simulink model "LazoAbierto_ConROS"  (R2021b)
settings: Solver=FixedStepAuto  StartTime=0.0  StopTime=8  FixedStep=T  RelTol=1e-3
undefined symbols (not defined in the file): fze, ModelName, Pose, ReferenceFrame, T, Twist
libraries: robotlib x13, robotcorelib x1
settings Model: Creator=carlo  LastModifiedBy=carlo
settings OptimizationCC: EnhancedBackFolding=on  PassReuseOutputArgsAs=Individual arguments  ZeroExternalMemoryAtStartup=off  ZeroInternalMemoryAtStartup=off  MaxStackSize=64  OptimizeBlockOrder=speed  DifferentSizesBufferReuse=on  OptimizationCustomize=off  EfficientTunableParamExpr=on
settings DebuggingCC: ParameterTunabilityLossMsg=error
settings HardwareCC: ProdBitPerLong=64  ProdHWDeviceType=Intel->x86-64 (Linux 64)  UseEmbeddedCoderFeatures=off
settings SFSimCC: MATLABDynamicMemAlloc=off
settings RTWCC: Description=Embedded Coder  SystemTargetFile=ert.tlc  HardwareBoard=Robot Operating System (ROS)  TLCOptions="-aInlineSetEventsForThisBaseRateFcn=TLC_FALSE -aSuppressMultiTaskScheduler=TLC_FALSE  -aRateBasedStepFcn=0"  TemplateMakefile=ert_default_tmf  Toolchain=Catkin  TargetLang=C++
settings CodeAppCC: ForceParamTrailComments=on  IgnoreCustomStorageClasses=off  OperatorAnnotations=on  SimulinkDataObjDesc=on  SFDataObjDesc=on  InsertBlockDesc=on
settings ERTTargetCC: SupportNonInlinedSFcns=on

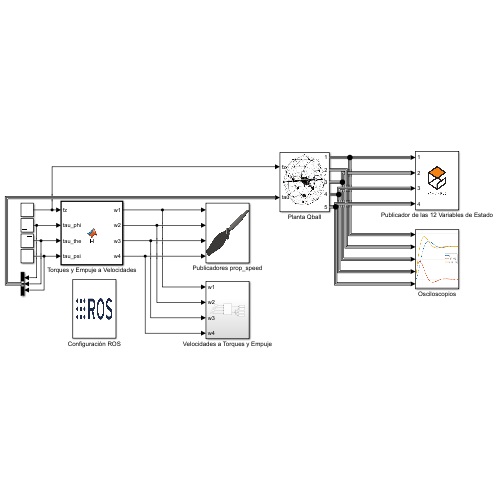
[thumbnail: Simulink's stored preview of the top-level diagram]
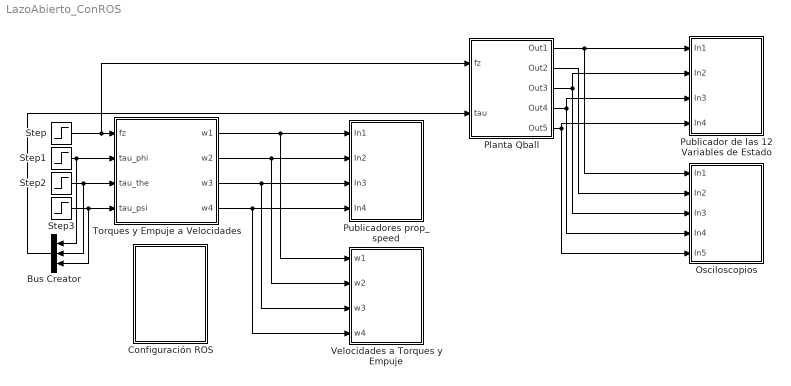
== system LazoAbierto_ConROS ==
  Bus Creator : BusCreator  Inputs=3
  Configuración ROS : Subsystem
      mask Display: image('$imagefile'); % Use "Edit Image" on toolstrip to change.
  Osciloscopios : Subsystem
      mask Display: image('C:\Users\carlo\OneDrive\Application Data\Escritorio\Tesis\Matlab\Imagenes\Osciloscopios.png'); % Use "Edit Image" on toolstrip to change.
  Planta Qball : Subsystem
      mask Display: image('$imagefile'); % Use "Edit Image" on toolstrip to change.
  Publicador de las 12 Variables de Estado : Subsystem
      mask Display: image('$imagefile'); % Use "Edit Image" on toolstrip to change.
  Publicadores prop_speed : Subsystem
      mask Display: image('$imagefile'); % Use "Edit Image" on toolstrip to change.
  Step : Step  Time=0  Before=fze+0.001  After=fze+0.001  SampleTime=0
  Step1 : Step  After=0  SampleTime=0
  Step2 : Step  After=0  SampleTime=0
  Step3 : Step  After=0  SampleTime=0
  Torques y Empuje a Velocidades : MATLAB Function  TreatAsAtomicUnit=on
  Velocidades a Torques y Empuje : Subsystem
  wires:
  Torques y Empuje a Velocidades/1(w1) -> Velocidades a Torques y Empuje/1(w1), Publicadores prop_speed/1(In1)
  Torques y Empuje a Velocidades/2(w2) -> Velocidades a Torques y Empuje/2(w2), Publicadores prop_speed/2(In2)
  Torques y Empuje a Velocidades/3(w3) -> Velocidades a Torques y Empuje/3(w3), Publicadores prop_speed/3(In3)
  Step/1 -> Planta Qball/1(fz), Torques y Empuje a Velocidades/1(fz)
  Step1/1 -> Bus Creator/1, Torques y Empuje a Velocidades/2(tau_phi)
  Step2/1 -> Bus Creator/2, Torques y Empuje a Velocidades/3(tau_the)
  Step3/1 -> Bus Creator/3, Torques y Empuje a Velocidades/4(tau_psi)
  Torques y Empuje a Velocidades/4(w4) -> Velocidades a Torques y Empuje/4(w4), Publicadores prop_speed/4(In4)
  Planta Qball/3(Out3) -> Publicador de las 12 Variables de Estado/2(In2), Osciloscopios/3(In3)
  Planta Qball/1(Out1) -> Publicador de las 12 Variables de Estado/1(In1), Osciloscopios/1(In1)
  Planta Qball/4(Out4) -> Publicador de las 12 Variables de Estado/3(In3), Osciloscopios/4(In4)
  Planta Qball/5(Out5) -> Publicador de las 12 Variables de Estado/4(In4), Osciloscopios/5(In5)
  Planta Qball/2(Out2) -> Osciloscopios/2(In2)
  Bus Creator/1 -> Planta Qball/2(tau)

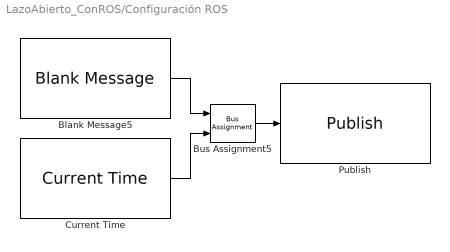
== system LazoAbierto_ConROS/Configuración ROS ==
  Blank Message5 : robotlib/Blank Message  messageClass=Message  entityType=rosgraph_msgs/Clock  messageType=rosgraph_msgs/Clock  SampleTime=inf  legacyBusStruct=off
  Bus Assignment5 : BusAssignment  AssignedSignals=Clock_
  Current Time : robotlib/Current Time  OutputFormat=bus  SampleTime=-1  ModelName=LazoAbierto_ConROS
      settings: SourceProductBaseCode=RR
  Publish : robotlib/Publish  topicSource=Select from ROS network  topic=/clock  messageType=rosgraph_msgs/Clock  legacyBusStruct=off  messageQueueLength=1
  wires:
  Blank Message5/1 -> Bus Assignment5/1
  Current Time/1 -> Bus Assignment5/2
  Bus Assignment5/1 -> Publish/1

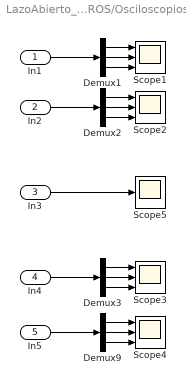
== system LazoAbierto_ConROS/Osciloscopios ==
  In1 : Inport
  In2 : Inport  Port=2
  In3 : Inport  Port=3
  In4 : Inport  Port=4
  In5 : Inport  Port=5
  Demux{1..3,9} (4 alike) : Demux  Outputs=3
  Scope{1..4} (4 alike) : Scope  NumInputPorts=3
  Scope5 : Scope
  wires:
  Demux3/2 -> Scope3/2
  Demux3/3 -> Scope3/3
  Demux9/1 -> Scope4/1
  Demux2/1 -> Scope2/1
  Demux3/1 -> Scope3/1
  Demux9/2 -> Scope4/2
  In4/1 -> Demux3/1
  Demux1/3 -> Scope1/3
  Demux1/1 -> Scope1/1
  Demux2/3 -> Scope2/3
  Demux1/2 -> Scope1/2
  Demux9/3 -> Scope4/3
  Demux2/2 -> Scope2/2
  In1/1 -> Demux1/1
  In5/1 -> Demux9/1
  In3/1 -> Scope5/1
  In2/1 -> Demux2/1

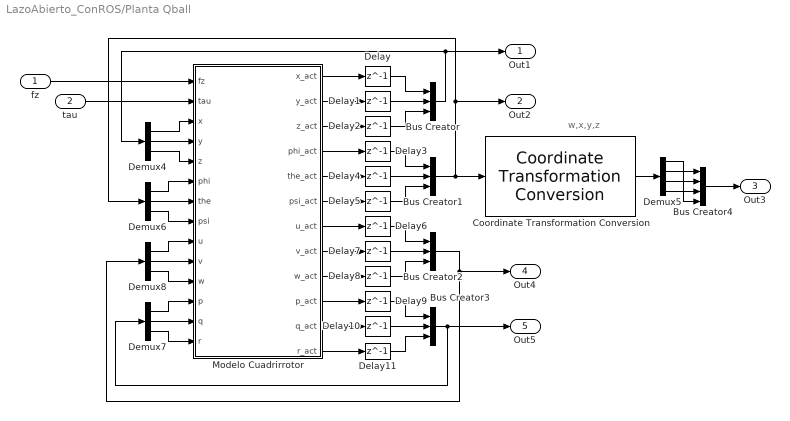
== system LazoAbierto_ConROS/Planta Qball ==
  note: w,x,y,z
  fz : Inport
  tau : Inport  Port=2
  Bus Creator{,1..3} (4 alike) : BusCreator  Inputs=3
  Bus Creator4 : BusCreator  Inputs=4
  Coordinate Transformation Conversion : robotcorelib/Coordinate Transformation Conversion  InputRepresentation=Euler Angles  InputEulerSequence=XYZ  ShowTrVecInputPort=on  OutputRepresentation=Quaternion  OutputEulerSequence=ZYX  ShowTrVecOutputPort=on  SimulateUsing=Interpreted execution
      settings: SourceProductBaseCode=NV,RO,RR,UV
  Delay{,1..11} (12 alike) : Delay  DelayLength=1  SampleTime=T
  Demux{4,6..8} (4 alike) : Demux  Outputs=3
  Demux5 : Demux
  Modelo Cuadrirrotor : MATLAB Function  TreatAsAtomicUnit=on
  Out1 : Outport
  Out2 : Outport  Port=2
  Out3 : Outport  Port=3
  Out4 : Outport  Port=4
  Out5 : Outport  Port=5
  wires:
  Modelo Cuadrirrotor/12(r_act) -> Delay11/1
  Modelo Cuadrirrotor/4(phi_act) -> Delay3/1
  Coordinate Transformation Conversion/1 -> Demux5/1
  Modelo Cuadrirrotor/5(the_act) -> Delay4/1
  Modelo Cuadrirrotor/1(x_act) -> Delay/1
  Delay4/1 -> Bus Creator1/2
  Bus Creator3/1 -> Out5/1, Demux7/1
  Delay/1 -> Bus Creator/1
  Bus Creator1/1 -> Out2/1, Demux6/1, Coordinate Transformation Conversion/1
  Demux4/1 -> Modelo Cuadrirrotor/3(x)
  Modelo Cuadrirrotor/9(w_act) -> Delay8/1
  Modelo Cuadrirrotor/7(u_act) -> Delay6/1
  Demux5/3 -> Bus Creator4/2
  Bus Creator2/1 -> Out4/1, Demux8/1
  Delay6/1 -> Bus Creator2/1
  Modelo Cuadrirrotor/6(psi_act) -> Delay5/1
  Modelo Cuadrirrotor/3(z_act) -> Delay2/1
  Modelo Cuadrirrotor/10(p_act) -> Delay9/1
  Bus Creator4/1 -> Out3/1
  Demux7/2 -> Modelo Cuadrirrotor/13(q)
  Delay11/1 -> Bus Creator3/3
  Delay5/1 -> Bus Creator1/3
  Delay9/1 -> Bus Creator3/1
  fz/1 -> Modelo Cuadrirrotor/1(fz)
  Delay2/1 -> Bus Creator/3
  Modelo Cuadrirrotor/8(v_act) -> Delay7/1
  Demux7/3 -> Modelo Cuadrirrotor/14(r)
  Delay7/1 -> Bus Creator2/2
  Demux7/1 -> Modelo Cuadrirrotor/12(p)
  Delay8/1 -> Bus Creator2/3
  Demux8/1 -> Modelo Cuadrirrotor/9(u)
  Bus Creator/1 -> Out1/1, Demux4/1
  Demux8/3 -> Modelo Cuadrirrotor/11(w)
  Demux5/2 -> Bus Creator4/1
  Delay1/1 -> Bus Creator/2
  Demux5/1 -> Bus Creator4/4
  Demux8/2 -> Modelo Cuadrirrotor/10(v)
  Demux4/2 -> Modelo Cuadrirrotor/4(y)
  Demux6/2 -> Modelo Cuadrirrotor/7(the)
  Demux6/3 -> Modelo Cuadrirrotor/8(psi)
  Demux4/3 -> Modelo Cuadrirrotor/5(z)
  Delay3/1 -> Bus Creator1/1
  Modelo Cuadrirrotor/2(y_act) -> Delay1/1
  Demux5/4 -> Bus Creator4/3
  Demux6/1 -> Modelo Cuadrirrotor/6(phi)
  Modelo Cuadrirrotor/11(q_act) -> Delay10/1
  Delay10/1 -> Bus Creator3/2
  tau/1 -> Modelo Cuadrirrotor/2(tau)

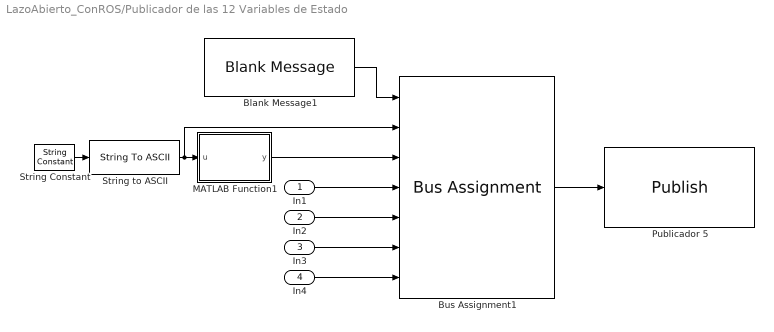
== system LazoAbierto_ConROS/Publicador de las 12 Variables de Estado ==
  In1 : Inport
  In2 : Inport  Port=2
  In3 : Inport  Port=3
  In4 : Inport  Port=4
  Blank Message1 : robotlib/Blank Message  messageClass=Message  entityType=gazebo_msgs/ModelState  messageType=gazebo_msgs/ModelState  SampleTime=inf  legacyBusStruct=off
  Bus Assignment1 : BusAssignment  AssignedSignals=ModelName,ReferenceFrame,Pose.Position,Pose.Orientation,Twist.Linear,Twist.Angular
  MATLAB Function1 : MATLAB Function  TreatAsAtomicUnit=on
  Publicador 5 : robotlib/Publish  topicSource=Specify your own  topic=/gazebo/model_state  messageType=gazebo_msgs/ModelState  legacyBusStruct=off  messageQueueLength=1
  String Constant : StringConstant  String="\"qball\""
  String to ASCII : StringToASCII  OutputVectorSize=128
  wires:
  String Constant/1 -> String to ASCII/1
  In4/1 -> Bus Assignment1/7
  Bus Assignment1/1 -> Publicador 5/1
  Blank Message1/1 -> Bus Assignment1/1
  In2/1 -> Bus Assignment1/5
  String to ASCII/1 -> Bus Assignment1/2, MATLAB Function1/1(u)
  MATLAB Function1/1(y) -> Bus Assignment1/3
  In3/1 -> Bus Assignment1/6
  In1/1 -> Bus Assignment1/4

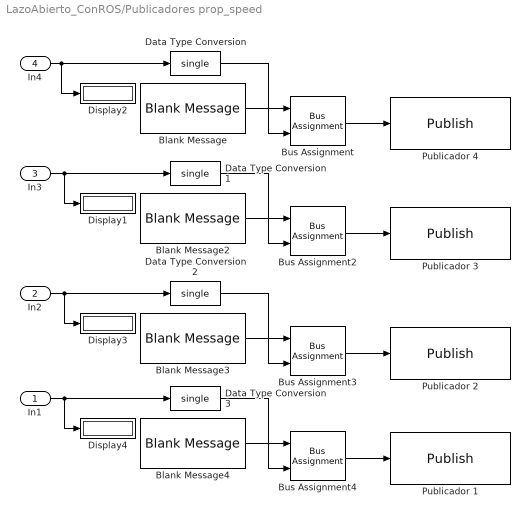
== system LazoAbierto_ConROS/Publicadores prop_speed ==
  In1 : Inport
  In2 : Inport  Port=2
  In3 : Inport  Port=3
  In4 : Inport  Port=4
  Blank Message{,2..4} (4 alike) : robotlib/Blank Message  messageClass=Message  entityType=std_msgs/Float32  messageType=std_msgs/Float32  SampleTime=inf  legacyBusStruct=off
  Bus Assignment{,2..4} (4 alike) : BusAssignment  AssignedSignals=Data
  Data Type Conversion{,1..3} (4 alike) : DataTypeConversion  OutDataTypeStr=single
  Display{1..4} (4 alike) : Display
  Publicador 1 : robotlib/Publish  topicSource=Specify your own  topic=/qball/prop1_speed  messageType=std_msgs/Float32  legacyBusStruct=off  messageQueueLength=1
  Publicador 2 : robotlib/Publish  topicSource=Specify your own  topic=/qball/prop2_speed  messageType=std_msgs/Float32  legacyBusStruct=off  messageQueueLength=1
  Publicador 3 : robotlib/Publish  topicSource=Specify your own  topic=/qball/prop3_speed  messageType=std_msgs/Float32  legacyBusStruct=off  messageQueueLength=1
  Publicador 4 : robotlib/Publish  topicSource=Specify your own  topic=/qball/prop4_speed  messageType=std_msgs/Float32  legacyBusStruct=off  messageQueueLength=1
  wires:
  Data Type Conversion/1 -> Bus Assignment/2
  Blank Message3/1 -> Bus Assignment3/1
  Bus Assignment/1 -> Publicador 4/1
  In4/1 -> Display2/1, Data Type Conversion/1
  Bus Assignment3/1 -> Publicador 2/1
  Data Type Conversion2/1 -> Bus Assignment3/2
  Blank Message/1 -> Bus Assignment/1
  Data Type Conversion1/1 -> Bus Assignment2/2
  Blank Message2/1 -> Bus Assignment2/1
  Bus Assignment2/1 -> Publicador 3/1
  Data Type Conversion3/1 -> Bus Assignment4/2
  Blank Message4/1 -> Bus Assignment4/1
  Bus Assignment4/1 -> Publicador 1/1
  In2/1 -> Display3/1, Data Type Conversion2/1
  In3/1 -> Display1/1, Data Type Conversion1/1
  In1/1 -> Data Type Conversion3/1, Display4/1

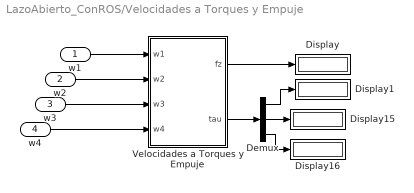
== system LazoAbierto_ConROS/Velocidades a Torques y Empuje ==
  w1 : Inport
  w2 : Inport  Port=2
  w3 : Inport  Port=3
  w4 : Inport  Port=4
  Demux : Demux  Outputs=3
  Display{,1,15..16} (4 alike) : Display
  Velocidades a Torques y Empuje : MATLAB Function  TreatAsAtomicUnit=on
  wires:
  Demux/3 -> Display16/1
  Velocidades a Torques y Empuje/1(fz) -> Display/1
  w2/1 -> Velocidades a Torques y Empuje/2(w2)
  Velocidades a Torques y Empuje/2(tau) -> Demux/1
  w1/1 -> Velocidades a Torques y Empuje/1(w1)
  Demux/1 -> Display1/1
  w3/1 -> Velocidades a Torques y Empuje/3(w3)
  Demux/2 -> Display15/1
  w4/1 -> Velocidades a Torques y Empuje/4(w4)

== matlab function LazoAbierto_ConROS/Publicador de las 12 Variables de Estado/MATLAB Function1 ==
  data: u input; y output
function y = fcn(u)

y = u';

== matlab function LazoAbierto_ConROS/Torques y Empuje a Velocidades ==
  data: fz input; w1 output; tau_phi input; w2 output; w3 output; w4 output; tau_the input; tau_psi input
function [w1,w2,w3,w4] = H(fz,tau_phi,tau_the,tau_psi)
%         Salidas          Entradas

% Constantes 
l = 0.2;    % m
kf = 0.007; % Nm/A
km = 0.8;   % V/kRPM

% Matriz H
H = [kf     kf      kf      kf;
     0      l*kf    0       -l*kf;
     -l*kf  0       l*kf    0;  
     km     -km     km      -km];
 
% Inversa de H
H_inversa = inv(H);

% Vector de entrada
Torques = [fz;
           tau_phi;
           tau_the;
           tau_psi];
       
% Vector de salida      
Wi2 = H_inversa * Torques;


% Velocidades angulares al cuadrado
w1 = sqrt(abs(Wi2(1)));
w2 = sqrt(abs(Wi2(2)));
w3 = sqrt(abs(Wi2(3)));
w4 = sqrt(abs(Wi2(4)));

== matlab function LazoAbierto_ConROS/Velocidades a Torques y Empuje/Velocidades a Torques y Empuje ==
  data: w1 input; fz output; w2 input; w3 input; w4 input; tau output

function [fz,tau] = H(w1,w2,w3,w4)
%         Salidas     Entradas

% wi rad/s

% Constantes
l = 0.2;    % m
kf = 0.007; % Nm/A
km = 0.8;   % V/kRPM

% Matriz H
H = [kf     kf      kf      kf;
     0      l*kf    0       -l*kf;
     -l*kf  0       l*kf    0;
     km     -km     km      -km];

Wi2 = [w1^2;
       w2^2;
       w3^2;
       w4^2];
 
Torques = H*Wi2;

fz = Torques(1);
tau_phi = Torques(2);
tau_the = Torques(3);
tau_psi = Torques(4);
tau = [tau_phi tau_the tau_psi];

== matlab function LazoAbierto_ConROS/Planta Qball/Modelo Cuadrirrotor ==
  data: x_act output; fz input; y_act output; tau input; z_act output; phi_act output; the_act output; psi_act output; u_act output; v_act output; w_act output; p_act output; q_act output; r_act output; x input; y input; z input; phi input; the input; psi input; u input; v input; w input; p input; q input; r input
function [x_act,y_act,z_act,phi_act,the_act,psi_act,u_act,v_act,w_act,p_act,q_act,r_act] ...
    = Cuadrirrotor(fz,tau,x,y,z,phi,the,psi,u,v,w,p,q,r)
%                  Salidas            Entradas 
                                  
%Constantes
m = 1.79;       g = 9.77412;
Ixx = 0.03;     Iyy = 0.03;
Izz = 0.04;     T = 0.01;


% Definición de los estados iniciales (dron en el piso y apagado)
%x = 0;     phi = 0;     u = 0;    p = 0;
%y = 0;     the = 0;     v = 0;    q = 0;
%z = 0;     psi = 0;     w = 0;    r = 0;   

 
d_x = u*cos(psi)*cos(the) - v*(cos(phi)*sin(psi) - sin(phi)*cos(psi)*sin(the))...
     + w*(sin(phi)*sin(psi) + cos(psi)*cos(phi)*sin(the));
d_y = u*cos(the)*sin(psi) + v*(cos(phi)*cos(psi) + sin(phi)*sin(psi)*sin(the))...
     - w*(cos(psi)*sin(phi) - cos(phi)*sin(psi)*sin(the));
d_z = -u*sin(the) + v*cos(the)*sin(phi) + w*cos(phi)*cos(the);

d_phi = p + q*sin(phi)*tan(the) + r*cos(phi)*tan(the);
d_the = q*cos(phi) - r*sin(phi);
d_psi = r*cos(phi)/cos(the) + q*sin(phi)/cos(the);

d_u = r*v - q*w - g*sin(the);
d_v = p*w - r*u + g*sin(phi)*cos(the);
d_w = q*u - p*v - fz/m + g*cos(phi)*cos(the);

d_p = (Iyy-Izz)/Ixx * q*r + tau(1)/Ixx;  
d_q = (Izz-Ixx)/Iyy * p*r - tau(2)/Iyy;
d_r = (Ixx-Iyy)/Izz * p*q - tau(3)/Izz;


% -------- Integración ----------------

% x_act = x_prev + T * d_x

x_act = x + T * d_x;
y_act = y + T * d_y;
z_act = (z + T * d_z); % Para invertir el eje z

phi_act = phi + T * d_phi;
the_act = the + T * d_the;
psi_act = psi + T * d_psi;

u_act = u + T * d_u;
v_act = v + T * d_v;
w_act = (w - T * d_w); % Para invertir el eje z  -+ mal

p_act = p + T * d_p;
q_act = q + T * d_q;
r_act = r + T * d_r;

end
